simulink model "RoboticsCoursework1"  (R2018b)
settings: Solver=ode4  StartTime=0.0  StopTime=5.0  RelTol=1e-3
undefined symbols (not defined in the file or in its folder): p560
libraries: roblocks x4
settings Model: Creator=57035  LastModifiedBy=57035

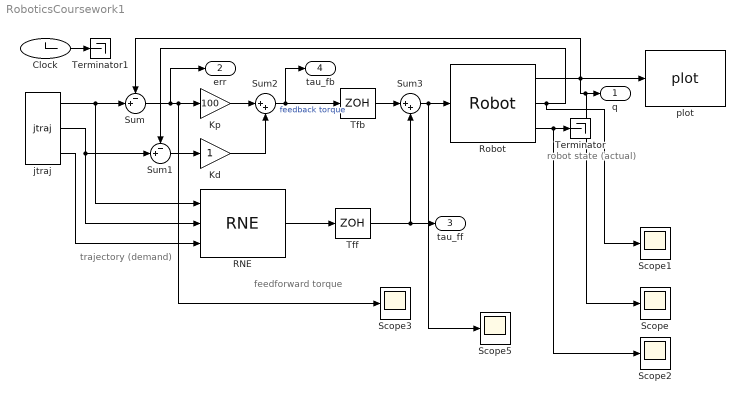
== system RoboticsCoursework1 ==
  note: feedforward torque
  note: trajectory
      | (demand)
  note: robot state
      | (actual)
  Clock : Clock
  Kd : Gain  SaturateOnIntegerOverflow=on  OutDataTypeStr=Inherit: Same as input  ParamDataTypeStr=Inherit: Same as input
  Kp : Gain  Gain=100  SaturateOnIntegerOverflow=on  OutDataTypeStr=Inherit: Same as input  ParamDataTypeStr=Inherit: Same as input
  RNE : roblocks/Dynamics/RNE  robot=p560.nofriction()  grav=[0 0 9.81]
  Robot : roblocks/Dynamics/Robot  robot=p560  q0=[3.2311 1.9518 0.0224 0 1.1674 -1.4813]*180/pi
  Scope{,1..3,5} (5 alike) : Scope
  Sum : Sum  Inputs=-+|  SaturateOnIntegerOverflow=on  InputSameDT=on  OutDataTypeStr=Inherit: Same as first input
  Sum1 : Sum  Inputs=-+|  SaturateOnIntegerOverflow=on  InputSameDT=on  OutDataTypeStr=Inherit: Same as first input
  Sum2 : Sum  Inputs=|++  SaturateOnIntegerOverflow=on  InputSameDT=on  OutDataTypeStr=Inherit: Same as first input
  Sum3 : Sum  Inputs=|++  SaturateOnIntegerOverflow=on  InputSameDT=on  OutDataTypeStr=Inherit: Same as first input
  Terminator : Terminator
  Terminator1 : Terminator
  Tfb : ZeroOrderHold  SampleTime=0.05
  Tff : ZeroOrderHold  SampleTime=0.05
  jtraj : roblocks/Trajectory/jtraj  q0=[3.2311 1.9518 0.0224 0 1.1674 -1.4813]*180/pi  qf=[3.5865 2.8632 -1.2022 1.6137 1.1278 -1.6707]*180/pi  tmax=2  ts=0.05
  plot : roblocks/Robot Graphics/plot  robot=p560  fps=25  holdplot=on
  q : Outport
  err : Outport  Port=2
  tau_ff : Outport  Port=3
  tau_fb : Outport  Port=4
  wires:
  Robot/3 -> Scope2/1, Terminator/1
  Clock/1 -> Terminator1/1
  Kp/1 -> Sum2/1
  Tff/1 -> Sum3/2, tau_ff/1
  Sum3/1 -> Scope5/1, Robot/1
  jtraj/3 -> RNE/3
  Robot/2 -> Scope1/1, Sum1/1
  jtraj/2 -> Sum1/2, RNE/2
  Kd/1 -> Sum2/2
  Robot/1 -> Scope/1, q/1, plot/1, Sum/1
  jtraj/1 -> RNE/1, Sum/2
  Sum/1 -> Scope3/1, Kp/1, err/1
  Tfb/1 -> Sum3/1
  Sum1/1 -> Kd/1
  Sum2/1 -> Tfb/1, tau_fb/1  "feedback torque"
  RNE/1 -> Tff/1
